simulink model "step_control"  (R2023a)
settings: Solver=VariableStepAuto  StartTime=0.0  StopTime=10.0  RelTol=1e-3
settings Model: Creator=HP  LastModifiedBy=HP

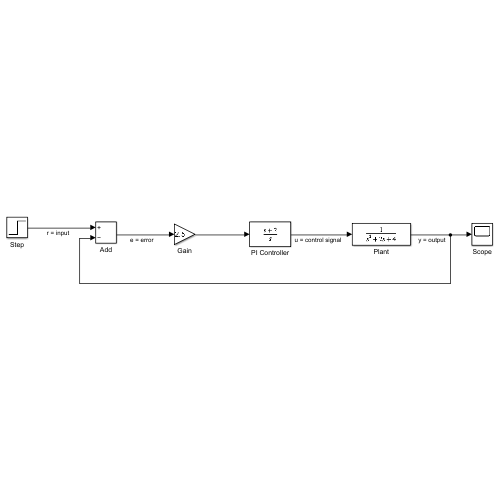
[thumbnail: Simulink's stored preview of the top-level diagram]
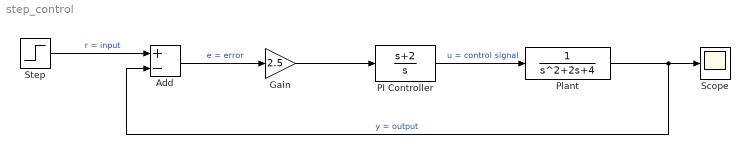
== system step_control ==
  Add : Sum  Inputs=+-
  Gain : Gain  Gain=2.5
  PI Controller : TransferFcn  Numerator=[1 2]  Denominator=[1 0]  ParameterTunability=Optimized
  Plant : TransferFcn  Denominator=[1 2 4]
  Scope : Scope
  Step : Step  SampleTime=0
  wires:
  Step/1 -> Add/1  "r = input"
  Add/1 -> Gain/1  "e = error"
  Gain/1 -> PI Controller/1
  PI Controller/1 -> Plant/1  "u = control signal"
  Plant/1 -> Add/2, Scope/1  "y = output"
